simulink model "Quaternions_Method_merge_main"  (R2021b)
settings: Solver=VariableStepAuto  StartTime=0.0  StopTime=Time  FixedStep=1e-1  RelTol=1e-13  AbsTol=1e-8
undefined symbols (not defined in the file or in its folder): a, A_BN_0, A_rw, A_rw_star, c, e, f_mag, H_0, i, magnitude, MB, mr, muP, omega_0, p_acc, RD, rho_d_MB, rho_s_MB, RS_MB, RS_SP, sig_b, sig_n, SP, T, t_sample, theta0, w_E
libraries: matrix_library x17, vrlib x8, simulink x2, simulink_extras x1
(part 6 of 6)

== system Quaternions_Method_merge_main/Enviroment/Solar Radiation Perturbation/Sum forces/determine highlighted area/creazione della matrice che ha per colonne i vettori distanza tra il CM del MB e i centri geom delle aree illuminate dal sole /creazione raggi vettore tra CM MB e centro facce illuminate della faccia che ha come normale l'asse j/If Action Subsystem6 ==
  Action Port : ActionPort  ActionPortLabel=else
  Constant : Constant  Value=[0;0;0]
  Out1 : Outport
  wires:
  Constant/1 -> Out1/1

== system Quaternions_Method_merge_main/Enviroment/Solar Radiation Perturbation/Sum forces/determine highlighted area/creazione della matrice che ha per colonne i vettori distanza tra il CM del MB e i centri geom delle aree illuminate dal sole /creazione raggi vettore tra CM MB e centro facce illuminate della faccia che ha come normale l'asse j/If Action Subsystem7 ==
  Action Port : ActionPort  ActionPortLabel=else
  Constant : Constant  Value=[0;0;0]
  Out1 : Outport
  wires:
  Constant/1 -> Out1/1

== system Quaternions_Method_merge_main/Enviroment/Solar Radiation Perturbation/Sum forces/determine highlighted area/creazione della matrice che ha per colonne i vettori distanza tra il CM del MB e i centri geom delle aree illuminate dal sole /creazione raggi vettore tra CM MB e centro facce illuminate della faccia che ha come normale l'asse j/creating distance between cm MB and centro geom lato1 ==
  MB : Inport
  Demux : Demux
  Ground : Ground
  Mux : Mux  Inputs=3
  Reshape : Reshape  OutputDimensionality=Column vector (2-D)
  Terminator : Terminator
  Terminator1 : Terminator
  Terminator2 : Terminator
  Out1 : Outport
  wires:
  Reshape/1 -> Out1/1
  Mux/1 -> Reshape/1
  Demux/4 -> Mux/3
  MB/1 -> Demux/1
  Demux/1 -> Terminator/1
  Demux/2 -> Terminator1/1
  Demux/3 -> Terminator2/1
  Ground/1 -> Mux/1, Mux/2

== system Quaternions_Method_merge_main/Enviroment/Solar Radiation Perturbation/Sum forces/determine highlighted area/creazione della matrice che ha per colonne i vettori distanza tra il CM del MB e i centri geom delle aree illuminate dal sole /creazione raggi vettore tra CM MB e centro facce illuminate della faccia che ha come normale l'asse k/If Action Subsystem ==
  Areas_vect : Inport
  MB : Inport  Port=2
  Action Port : ActionPort  ActionPortLabel=if(u1>0 & u2>0)
  Add : Sum  Inputs=+|-
  Add1 : Sum  Inputs=+|-
  Add2 : Sum
  Demux : Demux  Outputs=3
  Demux1 : Demux  Outputs=3
  Demux2 : Demux
  Divide : Product  Inputs=*/
  Divide1 : Product  Inputs=*/
  Gain{,1..3} (4 alike) : Gain  Gain=1/2
  Ground : Ground
  Ground1 : Ground
  Mux : Mux  Inputs=3
  Mux1 : Mux  Inputs=3
  Reshape{,1..3} (4 alike) : Reshape  OutputDimensionality=Column vector (2-D)
  Terminator{,1..3,8..9} (6 alike) : Terminator
  r_cface_cluce_xy_pos : Outport
  wires:
  Add/1 -> Mux/2
  Divide/1 -> Gain1/1
  Mux/1 -> Reshape2/1  "raggio vettore che collega il centro geom della faccia con il centro geom della faccia illuminata dal sole lungo j"
  Gain1/1 -> Add/2
  Demux/3 -> Divide/1
  [b_MB] -> Gain/1
  Gain/1 -> Add/1
  [a_MB] -> Divide/2
  Areas_vect/1 -> Reshape/1, Reshape1/1
  Ground1/1 -> Mux/1, Mux/3
  Reshape/1 -> Demux/1
  Add1/1 -> Mux1/1
  [b_MB] -> Divide1/2
  Mux1/1 -> Reshape3/1  "raggio vettore che collega il centro geom della faccia con il centro geom della faccia illuminata dal sole lungo x"
  Ground/1 -> Mux1/2, Mux1/3
  Demux1/3 -> Divide1/1
  Gain3/1 -> Add1/2
  Gain2/1 -> Add1/1
  Reshape1/1 -> Demux1/1
  Divide1/1 -> Gain3/1
  [a_MB] -> Gain2/1
  Reshape2/1 -> Add2/1
  Reshape3/1 -> Add2/2
  Add2/1 -> r_cface_cluce_xy_pos/1
  Demux1/1 -> Terminator/1
  Demux1/2 -> Terminator1/1
  Demux/1 -> Terminator9/1
  Demux/2 -> Terminator8/1
  MB/1 -> Demux2/1
  Demux2/1 -> Terminator2/1
  Demux2/2 -> [a_MB]
  Demux2/3 -> [b_MB]
  Demux2/4 -> Terminator3/1

== system Quaternions_Method_merge_main/Enviroment/Solar Radiation Perturbation/Sum forces/determine highlighted area/creazione della matrice che ha per colonne i vettori distanza tra il CM del MB e i centri geom delle aree illuminate dal sole /creazione raggi vettore tra CM MB e centro facce illuminate della faccia che ha come normale l'asse k/If Action Subsystem1 ==
  Areas_vect : Inport
  MB : Inport  Port=2
  Action Port : ActionPort  ActionPortLabel=if(u1>0 & u2<0)
  Add : Sum  Inputs=+|-
  Add1 : Sum  Inputs=+|-
  Add2 : Sum
  Demux : Demux  Outputs=3
  Demux1 : Demux  Outputs=3
  Demux2 : Demux
  Divide : Product  Inputs=*/
  Divide1 : Product  Inputs=*/
  Gain{,1..3} (4 alike) : Gain  Gain=1/2
  Gain4 : Gain  Gain=-1
  Ground : Ground
  Ground1 : Ground
  Mux : Mux  Inputs=3
  Mux1 : Mux  Inputs=3
  Reshape{,1..3} (4 alike) : Reshape  OutputDimensionality=Column vector (2-D)
  Terminator{,1..3,8..9} (6 alike) : Terminator
  r_cface_cluce_xpos_y_neg : Outport
  wires:
  Add/1 -> Gain4/1
  Divide/1 -> Gain1/1
  Mux/1 -> Reshape2/1  "raggio vettore che collega il centro geom della faccia con il centro geom della faccia illuminata dal sole lungo -j"
  Gain1/1 -> Add/2
  Demux/3 -> Divide/1
  Gain/1 -> Add/1
  Areas_vect/1 -> Reshape/1, Reshape1/1
  Ground1/1 -> Mux/1, Mux/3
  Reshape/1 -> Demux/1
  Mux1/1 -> Reshape3/1  "raggio vettore che collega il centro geom della faccia con il centro geom della faccia illuminata dal sole lungo i"
  Ground/1 -> Mux1/2, Mux1/3
  Demux1/3 -> Divide1/1
  Gain3/1 -> Add1/2
  Gain2/1 -> Add1/1
  Reshape1/1 -> Demux1/1
  Divide1/1 -> Gain3/1
  Reshape2/1 -> Add2/1
  Reshape3/1 -> Add2/2
  Add2/1 -> r_cface_cluce_xpos_y_neg/1
  Demux1/1 -> Terminator/1
  Demux1/2 -> Terminator1/1
  Demux/1 -> Terminator9/1
  Demux/2 -> Terminator8/1
  Gain4/1 -> Mux/2
  [a_MB] -> Divide/2
  [b_MB] -> Gain/1
  Add1/1 -> Mux1/1
  [b_MB] -> Divide1/2
  [a_MB] -> Gain2/1
  Demux2/1 -> Terminator2/1
  Demux2/2 -> [a_MB]
  MB/1 -> Demux2/1
  Demux2/3 -> [b_MB]
  Demux2/4 -> Terminator3/1

== system Quaternions_Method_merge_main/Enviroment/Solar Radiation Perturbation/Sum forces/determine highlighted area/creazione della matrice che ha per colonne i vettori distanza tra il CM del MB e i centri geom delle aree illuminate dal sole /creazione raggi vettore tra CM MB e centro facce illuminate della faccia che ha come normale l'asse k/If Action Subsystem2 ==
  Areas_vect : Inport
  MB1 : Inport  Port=2
  Action Port : ActionPort  ActionPortLabel=if(u1<0 & u2<0)
  Add : Sum  Inputs=+|-
  Add1 : Sum  Inputs=+|-
  Add2 : Sum
  Demux : Demux  Outputs=3
  Demux1 : Demux  Outputs=3
  Demux2 : Demux
  Divide : Product  Inputs=*/
  Divide1 : Product  Inputs=*/
  Gain{,1..3} (4 alike) : Gain  Gain=1/2
  Gain4 : Gain  Gain=-1
  Gain5 : Gain  Gain=-1
  Ground : Ground
  Ground1 : Ground
  Mux : Mux  Inputs=3
  Mux1 : Mux  Inputs=3
  Reshape{,1..3} (4 alike) : Reshape  OutputDimensionality=Column vector (2-D)
  Terminator{,1..3,8..9} (6 alike) : Terminator
  r_cface_cluce_xneg_y_neg : Outport
  wires:
  [a_MB] -> Divide1/2
  [b_MB] -> Gain2/1
  Add1/1 -> Gain5/1
  Gain4/1 -> Mux/1
  Add/1 -> Gain4/1
  [a_MB] -> Gain/1
  [b_MB] -> Divide/2
  Divide/1 -> Gain1/1
  Mux/1 -> Reshape2/1  "raggio vettore che collega il centro geom della faccia con il centro geom della faccia illuminata dal sole lungo -i"
  Gain1/1 -> Add/2
  Demux/3 -> Divide/1
  Gain/1 -> Add/1
  Areas_vect/1 -> Reshape/1, Reshape1/1
  Ground1/1 -> Mux/3, Mux/2
  Reshape/1 -> Demux/1
  Mux1/1 -> Reshape3/1  "raggio vettore che collega il centro geom della faccia con il centro geom della faccia illuminata dal sole lungo -j"
  Ground/1 -> Mux1/3, Mux1/1
  Demux1/3 -> Divide1/1
  Gain3/1 -> Add1/2
  Gain2/1 -> Add1/1
  Reshape1/1 -> Demux1/1
  Divide1/1 -> Gain3/1
  Reshape2/1 -> Add2/1
  Reshape3/1 -> Add2/2
  Add2/1 -> r_cface_cluce_xneg_y_neg/1
  Demux1/1 -> Terminator/1
  Demux1/2 -> Terminator1/1
  Demux/1 -> Terminator9/1
  Demux/2 -> Terminator8/1
  Gain5/1 -> Mux1/2
  Demux2/1 -> Terminator2/1
  Demux2/2 -> [a_MB]
  MB1/1 -> Demux2/1
  Demux2/3 -> [b_MB]
  Demux2/4 -> Terminator3/1

== system Quaternions_Method_merge_main/Enviroment/Solar Radiation Perturbation/Sum forces/determine highlighted area/creazione della matrice che ha per colonne i vettori distanza tra il CM del MB e i centri geom delle aree illuminate dal sole /creazione raggi vettore tra CM MB e centro facce illuminate della faccia che ha come normale l'asse k/If Action Subsystem3 ==
  Action Port : ActionPort  ActionPortLabel=else
  Constant : Constant  Value=[0;0;0]
  Out1 : Outport
  wires:
  Constant/1 -> Out1/1

== system Quaternions_Method_merge_main/Enviroment/Solar Radiation Perturbation/Sum forces/determine highlighted area/creazione della matrice che ha per colonne i vettori distanza tra il CM del MB e i centri geom delle aree illuminate dal sole /creazione raggi vettore tra CM MB e centro facce illuminate della faccia che ha come normale l'asse k/If Action Subsystem4 ==
  Areas_vect : Inport
  MB1 : Inport  Port=2
  Action Port : ActionPort  ActionPortLabel=if(u1<0 & u2>0)
  Add : Sum  Inputs=+|-
  Add1 : Sum  Inputs=+|-
  Add2 : Sum
  Demux : Demux  Outputs=3
  Demux1 : Demux  Outputs=3
  Demux2 : Demux
  Divide : Product  Inputs=*/
  Divide1 : Product  Inputs=*/
  Gain{,1..3} (4 alike) : Gain  Gain=1/2
  Gain4 : Gain  Gain=-1
  Ground : Ground
  Ground1 : Ground
  Mux : Mux  Inputs=3
  Mux1 : Mux  Inputs=3
  Reshape{,1..3} (4 alike) : Reshape  OutputDimensionality=Column vector (2-D)
  Terminator{,1..3,8..9} (6 alike) : Terminator
  r_cface_cluce_xneg_y_pos : Outport
  wires:
  Demux/2 -> Terminator8/1
  Demux/1 -> Terminator9/1
  Demux1/2 -> Terminator1/1
  Demux1/1 -> Terminator/1
  Add2/1 -> r_cface_cluce_xneg_y_pos/1
  Reshape3/1 -> Add2/2
  Reshape2/1 -> Add2/1
  Divide1/1 -> Gain3/1
  Reshape1/1 -> Demux1/1
  Gain2/1 -> Add1/1
  Gain3/1 -> Add1/2
  Demux1/3 -> Divide1/1
  Ground/1 -> Mux1/1, Mux1/3
  Mux1/1 -> Reshape3/1  "raggio vettore che collega il centro geom della faccia con il centro geom della faccia illuminata dal sole lungo j"
  Reshape/1 -> Demux/1
  Ground1/1 -> Mux/2, Mux/3
  Areas_vect/1 -> Reshape1/1, Reshape/1
  Gain/1 -> Add/1
  Demux/3 -> Divide/1
  Gain1/1 -> Add/2
  Mux/1 -> Reshape2/1  "raggio vettore che collega il centro geom della faccia con il centro geom della faccia illuminata dal sole lungo -i"
  Divide/1 -> Gain1/1
  [b_MB] -> Divide/2
  [a_MB] -> Gain/1
  Add/1 -> Gain4/1
  Gain4/1 -> Mux/1
  Add1/1 -> Mux1/2
  [b_MB] -> Gain2/1
  [a_MB] -> Divide1/2
  Demux2/1 -> Terminator2/1
  Demux2/2 -> [a_MB]
  MB1/1 -> Demux2/1
  Demux2/3 -> [b_MB]
  Demux2/4 -> Terminator3/1

== system Quaternions_Method_merge_main/Enviroment/Solar Radiation Perturbation/Sum forces/determine highlighted area/creazione della matrice che ha per colonne i vettori distanza tra il CM del MB e i centri geom delle aree illuminate dal sole /creazione raggi vettore tra CM MB e centro facce illuminate della faccia che ha come normale l'asse k/If Action Subsystem5 ==
  Action Port : ActionPort  ActionPortLabel=else
  Constant : Constant  Value=[0;0;0]
  Out1 : Outport
  wires:
  Constant/1 -> Out1/1

== system Quaternions_Method_merge_main/Enviroment/Solar Radiation Perturbation/Sum forces/determine highlighted area/creazione della matrice che ha per colonne i vettori distanza tra il CM del MB e i centri geom delle aree illuminate dal sole /creazione raggi vettore tra CM MB e centro facce illuminate della faccia che ha come normale l'asse k/If Action Subsystem6 ==
  Action Port : ActionPort  ActionPortLabel=else
  Constant : Constant  Value=[0;0;0]
  Out1 : Outport
  wires:
  Constant/1 -> Out1/1

== system Quaternions_Method_merge_main/Enviroment/Solar Radiation Perturbation/Sum forces/determine highlighted area/creazione della matrice che ha per colonne i vettori distanza tra il CM del MB e i centri geom delle aree illuminate dal sole /creazione raggi vettore tra CM MB e centro facce illuminate della faccia che ha come normale l'asse k/If Action Subsystem7 ==
  Action Port : ActionPort  ActionPortLabel=else
  Constant : Constant  Value=[0;0;0]
  Out1 : Outport
  wires:
  Constant/1 -> Out1/1

== system Quaternions_Method_merge_main/Enviroment/Solar Radiation Perturbation/Sum forces/determine highlighted area/creazione della matrice che ha per colonne i vettori distanza tra il CM del MB e i centri geom delle aree illuminate dal sole /creazione raggi vettore tra CM MB e centro facce illuminate della faccia che ha come normale l'asse k/creating distance between cm MB and centro geom lato1 ==
  MB : Inport
  Demux : Demux
  Ground : Ground
  Mux : Mux  Inputs=3
  Reshape : Reshape  OutputDimensionality=Column vector (2-D)
  Terminator : Terminator
  Terminator2 : Terminator
  Terminator3 : Terminator
  Out1 : Outport
  wires:
  Reshape/1 -> Out1/1
  Mux/1 -> Reshape/1
  MB/1 -> Demux/1
  Demux/1 -> Terminator/1
  Demux/2 -> Mux/1
  Demux/3 -> Terminator2/1
  Ground/1 -> Mux/2, Mux/3
  Demux/4 -> Terminator3/1

== matlab function Quaternions_Method_merge_main/Attitude determination/MATLAB Function ==
  data: K input; V output; D output
function [V, D] = fcn(K)
[V,D] = eig(K);
end

== matlab function Quaternions_Method_merge_main/Enviroment/Magnetic torque /Magnetic field in body frame/MATLAB Function ==
  data: R input; r_LVLH input; t input; teta input; B_N output
function B_N = fcn(R, r_LVLH, t, teta)

%% First thing is to define the vector containing all the polynimials up to the 4th order
P1 = 1;
P2 = teta;
P3 = ((3*teta^2)-1)/2;
P4 = ((5*teta^3)-(3*teta))/2;

% Computing the derivatives of the P polynomials
P1_der = 0;
P2_der = 1;
P3_der = 3*teta;
P4_der = ((15*teta^2)-3)/2;

r = norm(r_LVLH);
% Defining the order of the approximation k 
k = 4;

% Defining the matrices containing the coefficients needed to make the
% approximation model IGRF2000 (following the tables on the slide number 5 of the
% pack of slides number 8)
g = 1e9*[-29615 -1728 0 0 0; ...
                      -2267 3072 1672 0 0; ...
                     1341 -2290 1253 715 0; ...
                     935 787 251 -405 110]; %[T]
h = 1e9*[0 5186 0 0 0; ...
                     0 -2478 -458 0 0; ...
                     0 -227 296 -492 0; ...
                     0 272 -232 119 -304]; %[T]

% Computing the right ascension alpha, the declination delta, the longitude lon and the co-latitude phi
delta = asin(r_LVLH(3)/r); %[rad]
if(r_LVLH(2)/r > 0)
    alpha = acos((r_LVLH(1)/r)/cos(delta)); %[rad]
else 
    alpha = 2*pi -  acos((r_LVLH(1)/r)/cos(delta)); %[rad]
end
lat = -delta; %[rad]
phi = pi - lat; %[rad]
om_E = deg2rad(15.04)/3600; 
Gren_lon = om_E*t;
lon = (alpha - Gren_lon);

% Computing the for cicle to obtain components of B in r, th, phi RF
b_r = [];
b_th = [];
b_phi = [];
P_mat = [];
P_matder = [];
b1 = [];
b2 = [];
b3 = [];

syms v;
for n = 1:k
    P5 = (v^2-1)^n;
    Df1 = diff(P5,v,n);
    P_poly = 1/((2^n)*factorial(n))*Df1(teta);
    for m = 1:(n+1)
%         P_mat = (2*factorial(n-m))/factorial(n+m)*[P1, P1, P1, P1; P2, P2, P2, P2; P3, P3, P3, P3; P4, P4, P4, P4];
%         P_matder = ((2*factorial(n-m))/factorial(n+m))*[P1_der, P1_der, P1_der, P1_der; P2_der, P2_der, P2_der, P2_der; P3_der, P3_der, P3_der, P3_der; P4_der, P4_der, P4_der, P4_der];
%         b_r = (R/r)^n+2*(n+1)*((g(n, m)*cos(m*phi)+h(n,m)*sin(m*phi))*P_mat(n,m));
%         b_th = -(R/r)^(n+2)*((g(n, m)*cos(m*phi)+h(n,m)*sin(m*phi))*P_matder(n,m));
%         b_phi = -1/sin(teta)*((R/r)^(n+2))*((-g(n,m)*sin(m*phi) + h(n,m)*cos(m*phi))*P_mat(n,m));
          Df2 = diff(P_poly,v,m);
          Df3 = diff(P6,v, m);
          P6 = sqrt(((2*factorial(n-m))/factorial(n+m)))*((1-v^2)^1/(2*m))*Df2(teta);
          b_r = (R/r)^n+2*(n+1)*(g(n, m)*cos(m*phi)+h(n,m)*sin(m*phi))*sqrt(((2*factorial(n-m))/factorial(n+m)))*((1-v^2)^1/(2*m))*Df2(teta);
          b_th = -(R/r)^(n+2)*((g(n, m)*cos(m*phi)+h(n,m)*sin(m*phi))*P_matder(n,m))*Df3(teta);
          b_phi = -1/sin(teta)*((R/r)^(n+2))*((-g(n,m)*sin(m*phi) + h(n,m)*cos(m*phi))*P_mat(n,m))*sqrt(((2*factorial(n-m))/factorial(n+m)))*((1-v^2)^1/(2*m))*Df2(teta);

        % Computing the magnetic torque in the inertial frame 
        b1 = (b_r*cos(delta)+b_th*sin(delta))*cos(alpha)-b_phi*sin(alpha);
        b2 = (b_r*cos(delta)+b_th*sin(delta))*sin(alpha)+b_phi*cos(alpha);
        b3 = b_r*sin(delta)-b_th*cos(delta);
    end
end
B_N = [b1; b2; b3];


end
